simulink model "non_ideal_forward"  (R2018a)
settings: Solver=VariableStepAuto  StartTime=0.0  StopTime=0.02  MaxStep=1e-4  RelTol=1e-4  EnableMultiTasking=on
libraries: powerlib x22, simulink x1, powerlib_meascontrol x1
Description:
  | Copyright 2008-2018 The MathWorks, Inc.
settings Model: Creator=MathWorks  LastModifiedBy=HP
settings SolverCC: SolverResetMethod=Robust
settings DataIOCC: ReturnWorkspaceOutputs=on
settings OptimizationCC: LifeSpan=inf
settings DebuggingCC: ReadBeforeWriteMsg=DisableAll  WriteAfterWriteMsg=DisableAll  WriteAfterReadMsg=DisableAll  MultiTaskDSMMsg=none  SFUnexpectedBacktrackingDiag=warning  SFNoUnconditionalDefaultTransitionDiag=warning  SFExecutionAtInitializationDiag=none
settings ModelReferenceCC: UpdateModelReferenceTargets=IfOutOfDate
settings SFSimCC: SFSimEcho=off
settings CodeAppCC: StateflowObjectComments=on
settings GRTTargetCC: TargetLangStandard=C89/C90 (ANSI)  GeneratePreprocessorConditionals=Disable all
settings ConfigComp: CovMetricSettings=dw  CovHtmlReporting=on  CovSaveCumulativeToWorkspaceVar=on  CovSaveSingleToWorkspaceVar=on  CovExternalEMLEnable=off
settings SimscapeCC: SimscapeNormalizeSystem=off  SimscapeNominalValues={1, 'bar'; 1, 'cm^3/s'; 1, 'bar*kg/s'; 1, 'kJ/kg'; 1, 'kW'; }

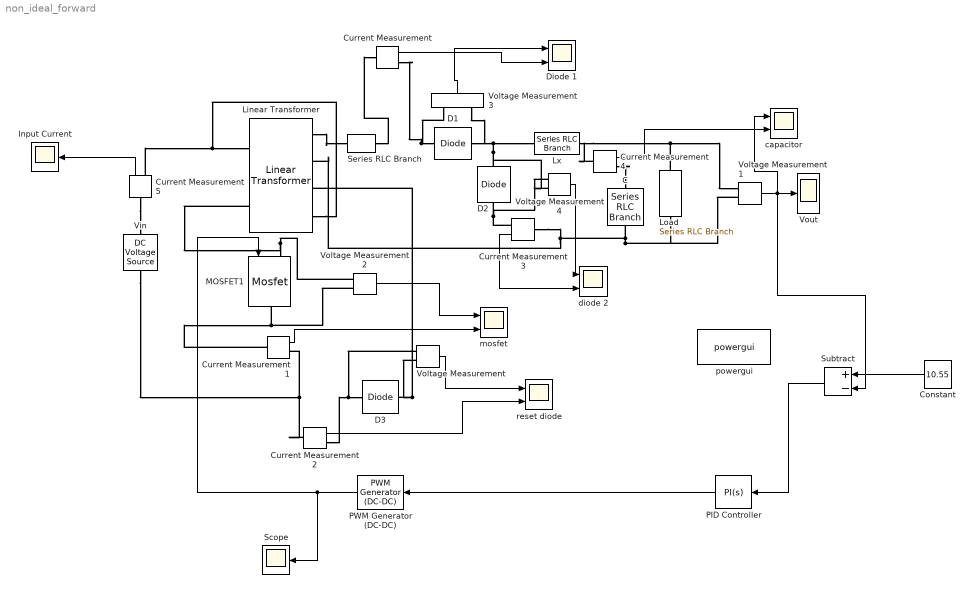
== system non_ideal_forward ==
  C : powerlib/Elements/Series RLC Branch  LConnTagsString=__new0  RConnTagsString=__new0  BranchType=RC  Resistance=40e-3  Inductance=200e-6  SetiL0=off  InitialCurrent=0  Capacitance=470e-6  Setx0=on  InitialVoltage=0  Measurements=None
  Constant : Constant  Value=10.55
  Current Measurement{,1..5} (6 alike) : powerlib/Measurements/Current Measurement  PhasorSimulation=off  OutputType=Complex  PSBequivalent=0
  D1 : powerlib/Power Electronics/Diode  Ron=1e-6  Lon=0  Vf=0.70  IC=0  UseSnubber=off  Rs=inf  Cs=0  Measurements=off
  D2 : powerlib/Power Electronics/Diode  Ron=1e-6  Lon=0  Vf=0.70  IC=0  UseSnubber=off  Rs=inf  Cs=0  Measurements=off
  D3 : powerlib/Power Electronics/Diode  Ron=1e-3  Lon=0  Vf=0.975  IC=0  UseSnubber=off  Rs=inf  Cs=0  Measurements=off
  Diode 1 : Scope  NumInputPorts=2
  Input Current : Scope
  Linear Transformer : powerlib/Elements/Linear Transformer  UNITS=SI  NominalPower=[ 50 100e3 ]  winding1=[54 5.123e-3 0]  winding2=[120 4.502e-3 0]  ThreeWindings=on  winding3=[54 0 0]  RmLm=[1e6 34.73e-3]  Measurements=Magnetization current  DataType=on
  Load : powerlib/Elements/Series RLC Branch  LConnTagsString=__new0  RConnTagsString=__new0  BranchType=R  Resistance=2.08  Inductance=200e-6  SetiL0=off  InitialCurrent=0  Capacitance=400e-6  Setx0=off  InitialVoltage=0  Measurements=Branch current
  Lx : powerlib/Elements/Series RLC Branch  LConnTagsString=__new0  RConnTagsString=__new0  BranchType=RL  Resistance=6.612e-3  Inductance=3.8e-3  SetiL0=off  InitialCurrent=0  Capacitance=400e-6  Setx0=off  InitialVoltage=0  Measurements=Branch current
  MOSFET1 : powerlib/Power Electronics/Mosfet  Ron=0.092  Lon=0  Rd=1e-3  Vfd=1.3  IC=0  Rs=1e6  Cs=inf  Measurements=off
  PID Controller : simulink/Continuous/PID Controller  Controller=PI  TimeDomain=Continuous-time  SampleTime=-1  IntegratorMethod=Forward Euler  FilterMethod=Forward Euler  Form=Parallel  UseFilter=on  ControllerParametersSource=internal  P=1  I=1  D=0  N=100  InitialConditionSource=internal  InitialConditionForIntegrator=0  InitialConditionForFilter=0  ExternalReset=none  LimitOutput=off  UpperSaturationLimit=inf  LowerSaturationLimit=-inf  LinearizeAsGain=on  AntiWindupMode=none  Kb=1  TrackingMode=off  Kt=1  PParamMin=[]  PParamMax=[]  IParamMin=[]  IParamMax=[]  DParamMin=[]  DParamMax=[]  NParamMin=[]  NParamMax=[]  KbParamMin=[]  KbParamMax=[]  KtParamMin=[]  KtParamMax=[]  POutMin=[]  POutMax=[]  IOutMin=[]  IOutMax=[]  DOutMin=[]  DOutMax=[]  NOutMin=[]  NOutMax=[]  KbOutMin=[]  KbOutMax=[]  KtOutMin=[]  KtOutMax=[]  IntegratorOutMin=[]  IntegratorOutMax=[]  FilterOutMin=[]  FilterOutMax=[]  SumOutMin=[]  SumOutMax=[]  SumI1OutMin=[]  SumI1OutMax=[]  SumI2OutMin=[]  SumI2OutMax=[]  SumI3OutMin=[]  SumI3OutMax=[]  SumDOutMin=[]  SumDOutMax=[]  SaturationOutMin=[]  SaturationOutMax=[]  IntegratorContinuousStateAttributes=''  IntegratorStateMustResolveToSignalObject=off  IntegratorRTWStateStorageClass=Auto  FilterContinuousStateAttributes=''  FilterStateMustResolveToSignalObject=off  FilterRTWStateStorageClass=Auto  DifferentiatorICPrevScaledInput=0  DifferentiatorOutMin=[]  DifferentiatorOutMax=[]  FilterDiffOutCoefMin=[]  FilterDiffOutCoefMax=[]  SumDenOutMin=[]  SumDenOutMax=[]  SumNumOutMin=[]  SumNumOutMax=[]  ReciprocalOutMin=[]  ReciprocalOutMax=[]  DivideOutMin=[]  DivideOutMax=[]  TunerSelectOption=Transfer Function Based (PID Tuner App)
  PWM Generator (DC-DC) : powerlib_meascontrol/Pulse & Signal Generators/PWM Generator (DC-DC)  Fsw=10000  Ts=0
  Scope : Scope
  Series RLC Branch : powerlib/Elements/Series RLC Branch  LConnTagsString=__new0  RConnTagsString=__new0  BranchType=L  Resistance=1  Inductance=34.73e-5  SetiL0=off  InitialCurrent=0  Capacitance=1e-6  Setx0=off  InitialVoltage=0  Measurements=None
  Subtract : Sum  Inputs=+-
  Vin : powerlib/Electrical Sources/DC Voltage Source  Amplitude=24  Measurements=None
  Voltage Measurement{,1..4} (5 alike) : powerlib/Measurements/Voltage Measurement  PhasorSimulation=off  OutputType=Complex  PSBequivalent=0
  Vout : Scope
  "capacitor " : Scope  NumInputPorts=2
  diode 2 : Scope  NumInputPorts=2
  mosfet : Scope  NumInputPorts=2
  powergui : powerlib/powergui  Priority=1  SimulationMode=Continuous  SampleTime=50e-6  frequency=60  Iterations=50  frequencyindice=0  Pbase=100e6  ErrMax=1e-4  UnitsV=kV  UnitsW=MW  buscounter=0  FunctionMessages=off  echomessages=off  EnableUseOfTLC=off  CurrentSourceSwitches=off  DisableSnubberDevices=off  DisableRonSwitches=off  DisableVfSwitches=off  DisplayEquations=off  SolverType=Tustin/Backward Euler (TBE)  Interpol=off  ExternalGateDelay=off  methode=off  Ts=100  x0status=blocks  SPID=on  SwTol=0  HookPort=off  RestoreLinks=warning  ResistiveCurrentMeasurement=off  Frange=[0:2:500]  Ylog=off  Xlog=on  ShowGrid=off  save=off  variable=ZData  structure=0  ZoomFFT=off  StartTime=0.0  cycles=1  DisplayStyle=1  fundamental=60  FreqAxis=off  MaxFrequency=1000  frequencyindicesteady=1  RmsSteady=1  display=off
  reset diode : Scope  NumInputPorts=2
  wires:
  Voltage Measurement1/1 -> "capacitor "/1, Subtract/2, Vout/1
  PWM Generator (DC-DC)/1 -> Scope/1, MOSFET1/1
  Constant/1 -> Subtract/1
  Subtract/1 -> PID Controller/1
  PID Controller/1 -> PWM Generator (DC-DC)/1
  Voltage Measurement2/1 -> mosfet/1
  Current Measurement1/1 -> mosfet/2
  Voltage Measurement/1 -> reset diode/1
  Current Measurement2/1 -> reset diode/2
  Voltage Measurement3/1 -> Diode 1/1
  Current Measurement/1 -> Diode 1/2
  Voltage Measurement4/1 -> diode 2/1
  Current Measurement3/1 -> diode 2/2
  Current Measurement4/1 -> "capacitor "/2
  Current Measurement5/1 -> Input Current/1
  connections:
  Load/LConn1 -- Current Measurement4/LConn1 -- Lx/RConn1 -- Voltage Measurement1/LConn1
  C/RConn1 -- Current Measurement3/LConn1 -- Linear Transformer/RConn2 -- Load/RConn1 -- Voltage Measurement1/LConn2
  Linear Transformer/LConn2 -- Voltage Measurement2/LConn1 -- MOSFET1/LConn1
  Voltage Measurement2/LConn2 -- Current Measurement1/LConn1 -- MOSFET1/RConn1
  Voltage Measurement3/LConn1 -- Current Measurement/RConn1 -- D1/LConn1
  Vin/LConn1 -- Current Measurement2/LConn1 -- Current Measurement1/RConn1
  Current Measurement2/RConn1 -- Voltage Measurement/LConn1 -- D3/LConn1
  Series RLC Branch/RConn1 -- Current Measurement/LConn1
  Current Measurement3/RConn1 -- Voltage Measurement4/LConn1 -- D2/LConn1
  Current Measurement4/RConn1 -- C/LConn1
  Linear Transformer/RConn4 -- Current Measurement5/RConn1 -- Linear Transformer/LConn1
  Linear Transformer/RConn1 -- Series RLC Branch/LConn1
  Voltage Measurement/LConn2 -- Linear Transformer/RConn3 -- D3/RConn1
  D2/RConn1 -- Voltage Measurement4/LConn2 -- Voltage Measurement3/LConn2 -- D1/RConn1 -- Lx/LConn1
  Current Measurement5/LConn1 -- Vin/RConn1
